simulink model "Jesse"  (R2023a)
settings: Solver=FixedStepDiscrete  StartTime=0.0  StopTime=60  FixedStep=0.01  RelTol=1e-3
undefined symbols (not defined in the file or in its folder): InputPWM, WheelSpeed
libraries: arduinolib x7, mobileRoboticsTrainingLib x1
settings Model: SimulationMode=external  ExtModeTrigDuration=2  Creator=Jack Youens  LastModifiedBy=ankus
settings OptimizationCC: EnhancedBackFolding=on  PassReuseOutputArgsAs=Individual arguments  ZeroExternalMemoryAtStartup=off  ZeroInternalMemoryAtStartup=off  MaxStackSize=64  OptimizeBlockOrder=speed  DifferentSizesBufferReuse=on  OptimizationCustomize=off  EfficientTunableParamExpr=on
settings DebuggingCC: ParameterTunabilityLossMsg=error
settings HardwareCC: ProdBitPerPointer=32  ProdBitPerSizeT=32  ProdBitPerPtrDiffT=32  ProdLargestAtomicInteger=Long  ProdLargestAtomicFloat=Double  ProdWordSize=32  ProdHWDeviceType=ARM Compatible->ARM Cortex
settings SFSimCC: MATLABDynamicMemAlloc=off
settings RTWCC: Description=Embedded Coder  SystemTargetFile=ert.tlc  HardwareBoard=Arduino Nano 33 IoT  TemplateMakefile=ert_default_tmf  Toolchain=Arduino ARM  BuildConfiguration=Faster Runs
settings CodeAppCC: ForceParamTrailComments=on  IgnoreCustomStorageClasses=off  OperatorAnnotations=on  SimulinkDataObjDesc=on  SFDataObjDesc=on  InsertBlockDesc=on
settings ERTTargetCC: SupportContinuousTime=on  SupportVariableSizeSignals=on  ExtModeTransport=3  ExtModeStaticAlloc=on  ExtModeAutomaticAllocSize=off  ExtModeStaticAllocSize=8192  ExtModeMexFile=ext_xcp  ExtModeIntrfLevel=Level2 - Open

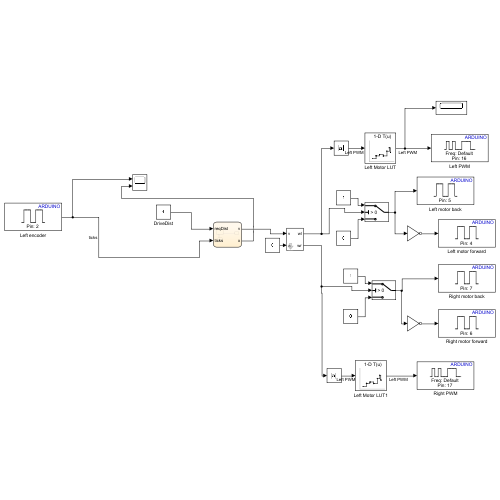
[thumbnail: Simulink's stored preview of the top-level diagram]
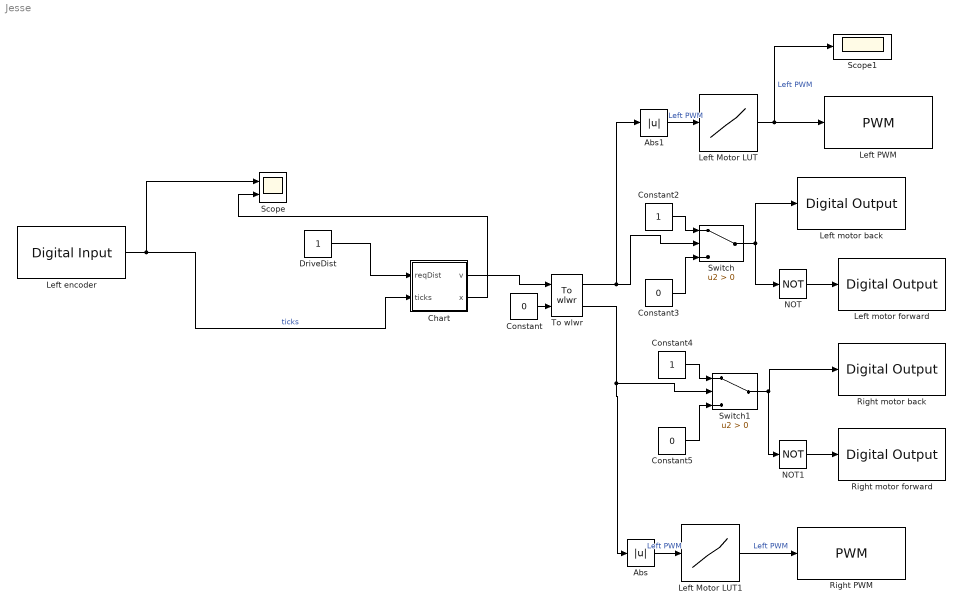
== system Jesse ==
  Abs : Abs  SaturateOnIntegerOverflow=off
  Abs1 : Abs  SaturateOnIntegerOverflow=off
  Chart : Stateflow chart  TreatAsAtomicUnit=on
  Constant : Constant  Value=0
  Constant2 : Constant
  Constant3 : Constant  Value=0
  Constant4 : Constant
  Constant5 : Constant  Value=0
  DriveDist : Constant
  Left Motor LUT : Lookup_n-D  NumberOfTableDimensions=1  BreakpointsForDimension1=WheelSpeed  Table=InputPWM  InterpMethod=Nearest  ExtrapMethod=Clip  InternalRulePriority=Speed  RndMeth=Simplest
  Left Motor LUT1 : Lookup_n-D  NumberOfTableDimensions=1  BreakpointsForDimension1=WheelSpeed  Table=InputPWM  InterpMethod=Nearest  ExtrapMethod=Clip  InternalRulePriority=Speed  RndMeth=Simplest
  Left PWM : arduinolib/PWM  pinNumber=16  frequencyType=Default  desiredFrequency=490.2  achievableFrequency=490.2
  Left encoder : arduinolib/Digital Input  pinNumber=2  mode=Default  Direction=input  SampleTime=0.1  blockPlatform=arduino
  Left motor back : arduinolib/Digital Output  pinNumber=5  Direction=output  blockPlatform=arduino
  Left motor forward : arduinolib/Digital Output  pinNumber=4  Direction=output  blockPlatform=arduino
  NOT : Logic  Operator=NOT  IconShape=distinctive  AllPortsSameDT=off  OutDataTypeStr=boolean
  NOT1 : Logic  Operator=NOT  IconShape=distinctive  AllPortsSameDT=off  OutDataTypeStr=boolean
  Right PWM : arduinolib/PWM  pinNumber=17  frequencyType=Default  desiredFrequency=490.2  achievableFrequency=490.2
  Right motor back : arduinolib/Digital Output  pinNumber=7  Direction=output  blockPlatform=arduino
  Right motor forward : arduinolib/Digital Output  pinNumber=6  Direction=output  blockPlatform=arduino
  Scope : Scope  NumInputPorts=2
  Scope1 : Scope
  Switch : Switch  Criteria=u2 > Threshold  SaturateOnIntegerOverflow=off  InputSameDT=off
  Switch1 : Switch  Criteria=u2 > Threshold  SaturateOnIntegerOverflow=off  InputSameDT=off
  To wlwr : mobileRoboticsTrainingLib/To wlwr  axleLength=axleLength  wheelR=wheelR
      link override change parameters: Gain=[1 -axleLength/2; 1 axleLength/2]
  wires:
  DriveDist/1 -> Chart/1(reqDist)
  Constant/1 -> To wlwr/2
  Left encoder/1 -> Chart/2(ticks), Scope/1  "ticks"
  To wlwr/1 -> Abs1/1, Switch/2
  Chart/2(x) -> Scope/2
  Abs1/1 -> Left Motor LUT/1  "Left PWM"
  Abs/1 -> Left Motor LUT1/1  "Left PWM"
  Constant2/1 -> Switch/1
  Constant3/1 -> Switch/3
  Switch/1 -> NOT/1, Left motor back/1
  NOT/1 -> Left motor forward/1
  Constant5/1 -> Switch1/3
  To wlwr/2 -> Abs/1, Switch1/2
  Constant4/1 -> Switch1/1
  Switch1/1 -> NOT1/1, Right motor back/1
  NOT1/1 -> Right motor forward/1
  Left Motor LUT/1 -> Scope1/1, Left PWM/1  "Left PWM"
  Left Motor LUT1/1 -> Right PWM/1  "Left PWM"
  Chart/1(v) -> To wlwr/1

== stateflow chart Jesse/Chart ==
  state Default
    entry:
    ticks;
    i;
    v=-10;
    dist1Tick=(pi*0.031)/10
    reqTicks=reqDist/dist1Tick;
  state Stop
    entry:
    v=0;
  state Move
    entry:
    v=-10;
    i=i+1;
    x=i;
  (default) -> Default
  Default -> Stop [order 2] : [i==reqTicks | i>reqTicks]
  Move -> Default
  Default -> Move [order 1] : [i<reqTicks && ticks==0]
  data: reqDist input; ticks input; v output; dist1Tick local; reqTicks local; i local =0; x output
